simulink model "set_nav420_to_NAVMODE_current_session_standalone_model"  (Simulink 7.4)
settings: Solver=ode3  StartTime=0.0  StopTime=inf  RelTol=1e-3
undefined symbols (not defined in the file or in its folder): serial
libraries: instrumentlib x2, NAV420Lib x1
settings Model: Creator=djulzz  LastModifiedBy=djulzz

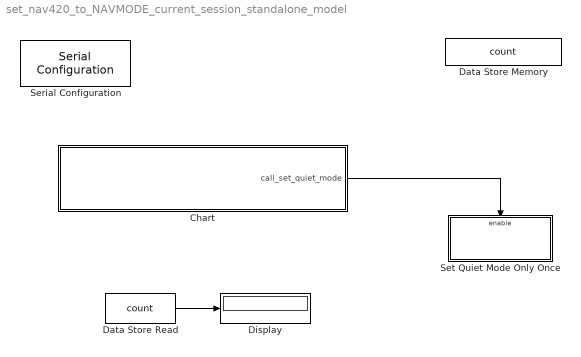
== system set_nav420_to_NAVMODE_current_session_standalone_model ==
  Chart : Stateflow chart
  Data Store Memory : DataStoreMemory  DataStoreName=count  DataType=uint8  OutDataType=fixdt(1, 16)  OutScaling=2^0  OutDataTypeStr=uint8
  Data Store Read : DataStoreRead  DataStoreName=count  SampleTime=-1
  Display : Display
      settings: Format=hex (Stored Integer)
  Serial Configuration : instrumentlib/Serial Configuration  Priority=-200000  DialogController=instrumentcreatedialog  DialogControllerArgs=DataTag0  ComPortMenu=COM1  ComPort=COM1  ObjConstructor=serial('COM1');  BaudRate=38400  DataBits=8  Parity=none  StopBits=1  FlowControl=none  Timeout=10  ByteOrder=LittleEndian
  Set Quiet Mode Only Once : Subsystem  TreatAsAtomicUnit=on
  wires:
  Data Store Read/1 -> Display/1
  Chart/1(call_set_quiet_mode) -> Set Quiet Mode Only Once/Enable

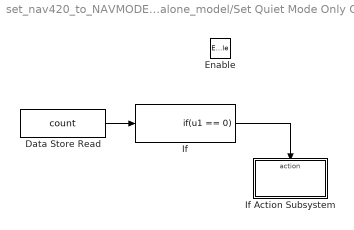
== system set_nav420_to_NAVMODE_current_session_standalone_model/Set Quiet Mode Only Once ==
  Enable : EnablePort
  Data Store Read : DataStoreRead  DataStoreName=count  SampleTime=-1
  If : If  IfExpression=u1 == 0  ShowElse=off
  If Action Subsystem : Subsystem  TreatAsAtomicUnit=on
  wires:
  Data Store Read/1 -> If/1
  If/1 -> If Action Subsystem/Action

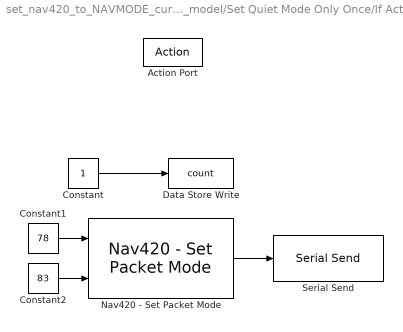
== system set_nav420_to_NAVMODE_current_session_standalone_model/Set Quiet Mode Only Once/If Action Subsystem ==
  Action Port : ActionPort  ActionType=then
  Constant : Constant  OutDataTypeMode=uint8  OutDataType=fixdt(1, 16)  OutScaling=2^0  OutDataTypeStr=uint8  SampleTime=-1
  Constant1 : Constant  Value=78  OutDataTypeMode=int8  OutDataType=fixdt(1, 16)  OutScaling=2^0  OutDataTypeStr=int8  SampleTime=-1
  Constant2 : Constant  Value=83  OutDataTypeMode=int8  OutDataType=fixdt(1, 16)  OutScaling=2^0  OutDataTypeStr=int8  SampleTime=-1
  Data Store Write : DataStoreWrite  DataStoreName=count  SampleTime=-1
  Nav420 - Set Packet Mode : NAV420Lib/Nav420 - Set Packet Mode  SystemSampleTime=-1
  Serial Send : instrumentlib/Serial Send  DialogController=instrumentcreatedialog  DialogControllerArgs=DataTag1  ComPortMenu=COM1  ComPort=COM1  ObjConstructor=serial('COM1');  Terminator=<none>  EnableBlockingMode=on
  wires:
  Constant/1 -> Data Store Write/1
  Constant2/1 -> Nav420 - Set Packet Mode/2
  Constant1/1 -> Nav420 - Set Packet Mode/1
  Nav420 - Set Packet Mode/1 -> Serial Send/1

== stateflow chart Chart ==
  state Step1
    count=0;
    call_set_quiet_mode=1;
  state End
  (default) -> Step1
  Step1 -> End
  data: count data_store_memory double; call_set_quiet_mode output uint8
